simulink model "gm_UZ_EnDat_be4_segregation"  (R2023b)
settings: Solver=FixedStepAuto  StartTime=0  StopTime=0.000505  RelTol=1e-3
model workspace (MAT data in the model file):
  Select = 0
libraries: hdlsllib x74, simulink x21, hdlmdlgenlib x4, simulink_extras x1
(part 2 of 5)

== system gm_UZ_EnDat_be4_segregation/UZ_ENDAT/CLKDIV7 ==
  CLK1 : Inport  OutDataTypeStr=boolean  PortDimensions=1  SampleTime=1e-08
  Delay : Delay  DelayLength=double(1)  InitialCondition=0  SampleTime=1e-08
  Logical Operator1 : Logic  Operator=NOT  Inputs=1  AllPortsSameDT=off  OutDataTypeStr=boolean  SampleTime=1e-08
  Triggered Subsystem : Subsystem
  CLK/2 : Outport  OutDataTypeStr=boolean  SampleTime=1e-08  VectorParamsAs1DForOutWhenUnconnected=off
  wires:
  Logical Operator1/1 -> CLK/2/1, Delay/1
  Triggered Subsystem/1(Q) -> Logical Operator1/1
  CLK1/1 -> Triggered Subsystem/2(Trigger)
  Delay/1 -> Triggered Subsystem/1(D)

== system gm_UZ_EnDat_be4_segregation/UZ_ENDAT/CLKDIV8 ==
  CLK1 : Inport  OutDataTypeStr=boolean  PortDimensions=1  SampleTime=1e-08
  Delay : Delay  DelayLength=double(1)  InitialCondition=0  SampleTime=1e-08
  Logical Operator1 : Logic  Operator=NOT  Inputs=1  AllPortsSameDT=off  OutDataTypeStr=boolean  SampleTime=1e-08
  Triggered Subsystem : Subsystem
  CLK/2 : Outport  OutDataTypeStr=boolean  SampleTime=1e-08  VectorParamsAs1DForOutWhenUnconnected=off
  wires:
  Logical Operator1/1 -> CLK/2/1, Delay/1
  Triggered Subsystem/1(Q) -> Logical Operator1/1
  CLK1/1 -> Triggered Subsystem/2(Trigger)
  Delay/1 -> Triggered Subsystem/1(D)

== system gm_UZ_EnDat_be4_segregation/UZ_ENDAT/CLKDIV9 ==
  CLK1 : Inport  OutDataTypeStr=boolean  PortDimensions=1  SampleTime=1e-08
  Delay : Delay  DelayLength=double(1)  InitialCondition=0  SampleTime=1e-08
  Logical Operator1 : Logic  Operator=NOT  Inputs=1  AllPortsSameDT=off  OutDataTypeStr=boolean  SampleTime=1e-08
  Triggered Subsystem : Subsystem
  CLK/2 : Outport  OutDataTypeStr=boolean  SampleTime=1e-08  VectorParamsAs1DForOutWhenUnconnected=off
  wires:
  Logical Operator1/1 -> CLK/2/1, Delay/1
  Triggered Subsystem/1(Q) -> Logical Operator1/1
  CLK1/1 -> Triggered Subsystem/2(Trigger)
  Delay/1 -> Triggered Subsystem/1(D)

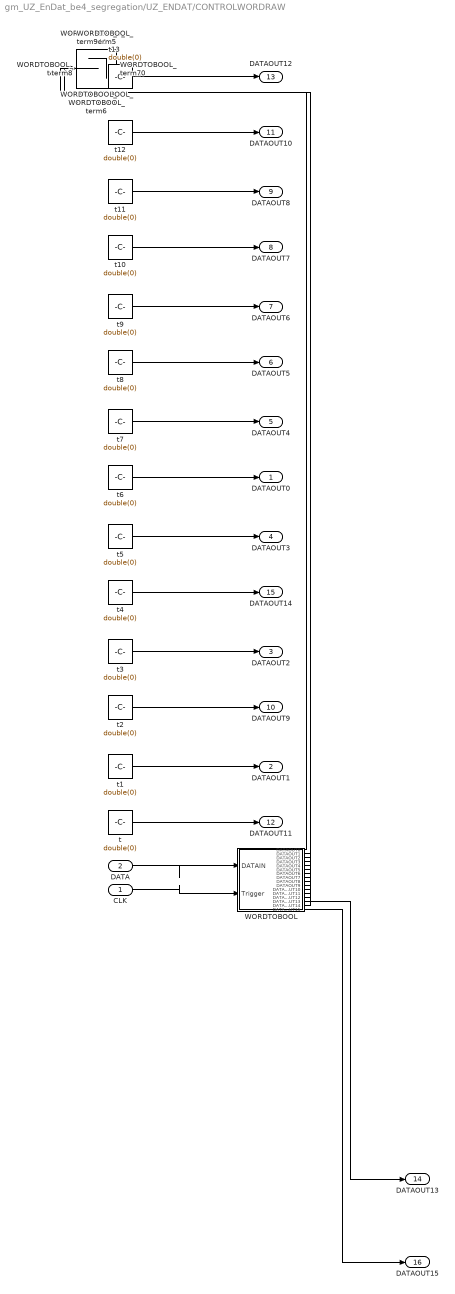
== system gm_UZ_EnDat_be4_segregation/UZ_ENDAT/CONTROLWORDRAW ==
  CLK : Inport  OutDataTypeStr=boolean  PortDimensions=1  SampleTime=1e-08
  DATA : Inport  Port=2  OutDataTypeStr=uint16  PortDimensions=1  SampleTime=1e-08
  WORDTOBOOL : Subsystem
  WORDTOBOOL_term{0..12,14} (14 alike) : Terminator
  t{,1..13} (14 alike) : Constant  Value=double(0)  OutDataTypeStr=boolean  SampleTime=1e-08
  DATAOUT0 : Outport  SampleTime=1e-08  VectorParamsAs1DForOutWhenUnconnected=off
  DATAOUT1 : Outport  Port=2  SampleTime=1e-08  VectorParamsAs1DForOutWhenUnconnected=off
  DATAOUT2 : Outport  Port=3  SampleTime=1e-08  VectorParamsAs1DForOutWhenUnconnected=off
  DATAOUT3 : Outport  Port=4  SampleTime=1e-08  VectorParamsAs1DForOutWhenUnconnected=off
  DATAOUT4 : Outport  Port=5  SampleTime=1e-08  VectorParamsAs1DForOutWhenUnconnected=off
  DATAOUT5 : Outport  Port=6  SampleTime=1e-08  VectorParamsAs1DForOutWhenUnconnected=off
  DATAOUT6 : Outport  Port=7  SampleTime=1e-08  VectorParamsAs1DForOutWhenUnconnected=off
  DATAOUT7 : Outport  Port=8  SampleTime=1e-08  VectorParamsAs1DForOutWhenUnconnected=off
  DATAOUT8 : Outport  Port=9  SampleTime=1e-08  VectorParamsAs1DForOutWhenUnconnected=off
  DATAOUT9 : Outport  Port=10  SampleTime=1e-08  VectorParamsAs1DForOutWhenUnconnected=off
  DATAOUT10 : Outport  Port=11  SampleTime=1e-08  VectorParamsAs1DForOutWhenUnconnected=off
  DATAOUT11 : Outport  Port=12  SampleTime=1e-08  VectorParamsAs1DForOutWhenUnconnected=off
  DATAOUT12 : Outport  Port=13  SampleTime=1e-08  VectorParamsAs1DForOutWhenUnconnected=off
  DATAOUT13 : Outport  Port=14  SampleTime=1e-08  VectorParamsAs1DForOutWhenUnconnected=off
  DATAOUT14 : Outport  Port=15  SampleTime=1e-08  VectorParamsAs1DForOutWhenUnconnected=off
  DATAOUT15 : Outport  Port=16  SampleTime=1e-08  VectorParamsAs1DForOutWhenUnconnected=off
  wires:
  CLK/1 -> WORDTOBOOL/2(Trigger)
  DATA/1 -> WORDTOBOOL/1(DATAIN)
  t6/1 -> DATAOUT0/1
  t1/1 -> DATAOUT1/1
  t3/1 -> DATAOUT2/1
  t5/1 -> DATAOUT3/1
  t7/1 -> DATAOUT4/1
  t8/1 -> DATAOUT5/1
  t9/1 -> DATAOUT6/1
  t10/1 -> DATAOUT7/1
  t11/1 -> DATAOUT8/1
  t2/1 -> DATAOUT9/1
  t12/1 -> DATAOUT10/1
  t/1 -> DATAOUT11/1
  t13/1 -> DATAOUT12/1
  WORDTOBOOL/14(DATAOUT13) -> DATAOUT13/1
  t4/1 -> DATAOUT14/1
  WORDTOBOOL/16(DATAOUT15) -> DATAOUT15/1
  WORDTOBOOL/1(DATAOUT0) -> WORDTOBOOL_term0/1
  WORDTOBOOL/2(DATAOUT1) -> WORDTOBOOL_term1/1
  WORDTOBOOL/3(DATAOUT2) -> WORDTOBOOL_term2/1
  WORDTOBOOL/4(DATAOUT3) -> WORDTOBOOL_term3/1
  WORDTOBOOL/5(DATAOUT4) -> WORDTOBOOL_term4/1
  WORDTOBOOL/6(DATAOUT5) -> WORDTOBOOL_term5/1
  WORDTOBOOL/7(DATAOUT6) -> WORDTOBOOL_term6/1
  WORDTOBOOL/8(DATAOUT7) -> WORDTOBOOL_term7/1
  WORDTOBOOL/9(DATAOUT8) -> WORDTOBOOL_term8/1
  WORDTOBOOL/10(DATAOUT9) -> WORDTOBOOL_term9/1
  WORDTOBOOL/11(DATAOUT10) -> WORDTOBOOL_term10/1
  WORDTOBOOL/12(DATAOUT11) -> WORDTOBOOL_term11/1
  WORDTOBOOL/13(DATAOUT12) -> WORDTOBOOL_term12/1
  WORDTOBOOL/15(DATAOUT14) -> WORDTOBOOL_term14/1

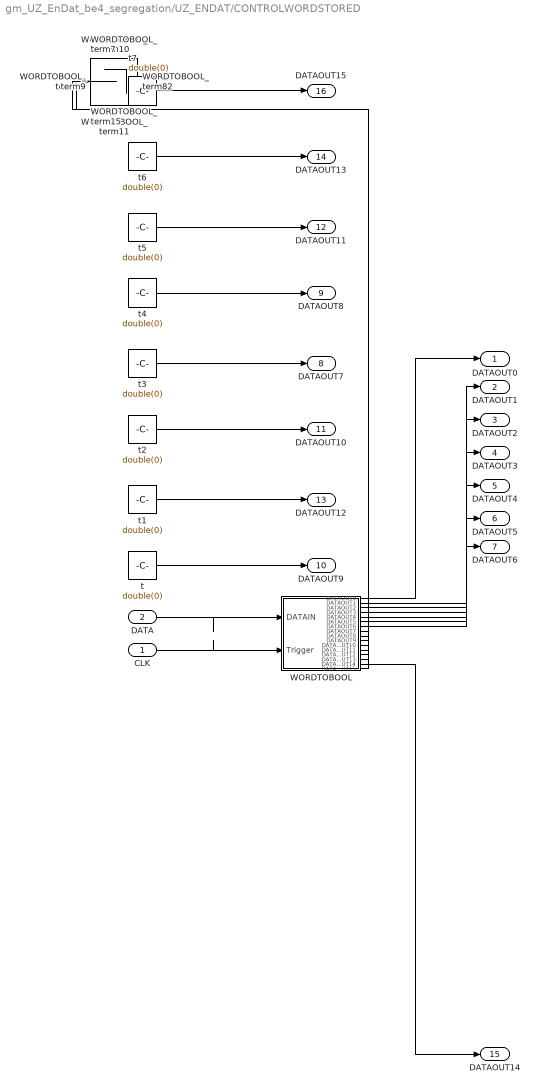
== system gm_UZ_EnDat_be4_segregation/UZ_ENDAT/CONTROLWORDSTORED ==
  CLK : Inport  OutDataTypeStr=boolean  PortDimensions=1  SampleTime=1e-08
  DATA : Inport  Port=2  OutDataTypeStr=uint16  PortDimensions=1  SampleTime=1e-08
  WORDTOBOOL : Subsystem
  WORDTOBOOL_term{7..13,15} (8 alike) : Terminator
  t{,1..7} (8 alike) : Constant  Value=double(0)  OutDataTypeStr=boolean  SampleTime=1e-08
  DATAOUT0 : Outport  SampleTime=1e-08  VectorParamsAs1DForOutWhenUnconnected=off
  DATAOUT1 : Outport  Port=2  SampleTime=1e-08  VectorParamsAs1DForOutWhenUnconnected=off
  DATAOUT2 : Outport  Port=3  SampleTime=1e-08  VectorParamsAs1DForOutWhenUnconnected=off
  DATAOUT3 : Outport  Port=4  SampleTime=1e-08  VectorParamsAs1DForOutWhenUnconnected=off
  DATAOUT4 : Outport  Port=5  SampleTime=1e-08  VectorParamsAs1DForOutWhenUnconnected=off
  DATAOUT5 : Outport  Port=6  SampleTime=1e-08  VectorParamsAs1DForOutWhenUnconnected=off
  DATAOUT6 : Outport  Port=7  SampleTime=1e-08  VectorParamsAs1DForOutWhenUnconnected=off
  DATAOUT7 : Outport  Port=8  SampleTime=1e-08  VectorParamsAs1DForOutWhenUnconnected=off
  DATAOUT8 : Outport  Port=9  SampleTime=1e-08  VectorParamsAs1DForOutWhenUnconnected=off
  DATAOUT9 : Outport  Port=10  SampleTime=1e-08  VectorParamsAs1DForOutWhenUnconnected=off
  DATAOUT10 : Outport  Port=11  SampleTime=1e-08  VectorParamsAs1DForOutWhenUnconnected=off
  DATAOUT11 : Outport  Port=12  SampleTime=1e-08  VectorParamsAs1DForOutWhenUnconnected=off
  DATAOUT12 : Outport  Port=13  SampleTime=1e-08  VectorParamsAs1DForOutWhenUnconnected=off
  DATAOUT13 : Outport  Port=14  SampleTime=1e-08  VectorParamsAs1DForOutWhenUnconnected=off
  DATAOUT14 : Outport  Port=15  SampleTime=1e-08  VectorParamsAs1DForOutWhenUnconnected=off
  DATAOUT15 : Outport  Port=16  SampleTime=1e-08  VectorParamsAs1DForOutWhenUnconnected=off
  wires:
  CLK/1 -> WORDTOBOOL/2(Trigger)
  DATA/1 -> WORDTOBOOL/1(DATAIN)
  WORDTOBOOL/1(DATAOUT0) -> DATAOUT0/1
  WORDTOBOOL/2(DATAOUT1) -> DATAOUT1/1
  WORDTOBOOL/3(DATAOUT2) -> DATAOUT2/1
  WORDTOBOOL/4(DATAOUT3) -> DATAOUT3/1
  WORDTOBOOL/5(DATAOUT4) -> DATAOUT4/1
  WORDTOBOOL/6(DATAOUT5) -> DATAOUT5/1
  WORDTOBOOL/7(DATAOUT6) -> DATAOUT6/1
  t3/1 -> DATAOUT7/1
  t4/1 -> DATAOUT8/1
  t/1 -> DATAOUT9/1
  t2/1 -> DATAOUT10/1
  t5/1 -> DATAOUT11/1
  t1/1 -> DATAOUT12/1
  t6/1 -> DATAOUT13/1
  WORDTOBOOL/15(DATAOUT14) -> DATAOUT14/1
  t7/1 -> DATAOUT15/1
  WORDTOBOOL/8(DATAOUT7) -> WORDTOBOOL_term7/1
  WORDTOBOOL/9(DATAOUT8) -> WORDTOBOOL_term8/1
  WORDTOBOOL/10(DATAOUT9) -> WORDTOBOOL_term9/1
  WORDTOBOOL/11(DATAOUT10) -> WORDTOBOOL_term10/1
  WORDTOBOOL/12(DATAOUT11) -> WORDTOBOOL_term11/1
  WORDTOBOOL/13(DATAOUT12) -> WORDTOBOOL_term12/1
  WORDTOBOOL/14(DATAOUT13) -> WORDTOBOOL_term13/1
  WORDTOBOOL/16(DATAOUT15) -> WORDTOBOOL_term15/1

== system gm_UZ_EnDat_be4_segregation/UZ_ENDAT/CRC_Check ==
  data : Inport  OutDataTypeStr=boolean  PortDimensions=1  SampleTime=1e-08
  set : Inport  Port=2  OutDataTypeStr=boolean  PortDimensions=1  SampleTime=1e-08
  clk : Inport  Port=3  OutDataTypeStr=boolean  PortDimensions=1  SampleTime=1e-08
  Constant : Constant  OutDataTypeStr=boolean  SampleTime=1e-08
  Constant1 : Constant  Value=0  OutDataTypeStr=boolean  SampleTime=1e-08
  FF0 : Subsystem
  FF0_term1 : Terminator
  FF1 : Subsystem
  FF1_term1 : Terminator
  FF2 : Subsystem
  FF2_term1 : Terminator
  FF3 : Subsystem
  FF3_term1 : Terminator
  FF4 : Subsystem
  Logical Operator : Logic  Operator=OR  AllPortsSameDT=off  OutDataTypeStr=boolean  SampleTime=1e-08
  Logical Operator{1..2,5..6} (4 alike) : Logic  AllPortsSameDT=off  OutDataTypeStr=boolean  SampleTime=1e-08
  Logical Operator3 : Logic  Operator=NOT  Inputs=1  AllPortsSameDT=off  OutDataTypeStr=boolean  SampleTime=1e-08
  Logical Operator4 : Logic  Operator=NOT  Inputs=1  AllPortsSameDT=off  OutDataTypeStr=boolean  SampleTime=1e-08
  Memory : UnitDelay  SampleTime=1e-08
  Memory1 : UnitDelay  SampleTime=1e-08
  Relational Operator : RelationalOperator  Operator===  OutDataTypeStr=boolean  SampleTime=1e-08  InputSameDT=off
  Relational Operator1 : RelationalOperator  Operator===  OutDataTypeStr=boolean  SampleTime=1e-08  InputSameDT=off
  Relational Operator2 : RelationalOperator  Operator===  OutDataTypeStr=boolean  SampleTime=1e-08  InputSameDT=off
  crc : Outport  SampleTime=1e-08
  wires:
  data/1 -> Logical Operator1/1, Relational Operator/2
  set/1 -> Logical Operator4/1, Logical Operator5/2, Logical Operator6/2
  clk/1 -> FF1/2(CLK), FF2/2(CLK), FF3/2(CLK), FF4/2(CLK), FF0/2(CLK)
  Constant/1 -> FF1/1(S), FF2/1(S), FF3/1(S), FF4/1(S), FF0/1(S)
  Constant1/1 -> FF1/4(R), FF2/4(R), FF3/4(R), FF4/4(R), FF0/4(R)
  FF0/2(NQ) -> FF0_term1/1
  FF1/2(NQ) -> FF1_term1/1
  FF2/2(NQ) -> FF2_term1/1
  FF3/2(NQ) -> FF3_term1/1
  FF4/2(NQ) -> Logical Operator2/1
  Logical Operator/1 -> crc/1
  Logical Operator1/1 -> Logical Operator/1
  Logical Operator2/1 -> Logical Operator/2
  Logical Operator3/1 -> Logical Operator1/2
  Logical Operator4/1 -> Logical Operator3/1, Logical Operator2/2
  Memory/1 -> Relational Operator1/2, Relational Operator2/2
  Logical Operator5/1 -> Memory1/1
  FF4/1(Q) -> Logical Operator5/1
  Logical Operator6/1 -> Memory/1
  Relational Operator/1 -> FF0/3(DATA), Logical Operator6/1
  Memory1/1 -> Relational Operator/1
  Relational Operator1/1 -> FF1/3(DATA)
  FF0/1(Q) -> Relational Operator1/1
  FF1/1(Q) -> FF2/3(DATA)
  Relational Operator2/1 -> FF3/3(DATA)
  FF2/1(Q) -> Relational Operator2/1
  FF3/1(Q) -> FF4/3(DATA)

== system gm_UZ_EnDat_be4_segregation/UZ_ENDAT/Compare To Constant ==
  u : Inport  OutDataTypeStr=fixdt(0,4,0,'DataTypeOverride', 'Off')  SampleTime=1e-08
  Compare : RelationalOperator  Operator===  OutDataTypeStr=boolean
  Constant : Constant  DisableCoverage=on  Value=const  OutDataTypeStr=Inherit: Inherit via back propagation  SampleTime=-1
  y : Outport  SampleTime=1e-08
  wires:
  u/1 -> Compare/1
  Compare/1 -> y/1
  Constant/1 -> Compare/2

== system gm_UZ_EnDat_be4_segregation/UZ_ENDAT/Compare To Constant1 ==
  u : Inport  OutDataTypeStr=fixdt(0,4,0,'DataTypeOverride', 'Off')  SampleTime=1e-08
  Compare : RelationalOperator  Operator===  OutDataTypeStr=boolean
  Constant : Constant  DisableCoverage=on  Value=const  OutDataTypeStr=Inherit: Inherit via back propagation  SampleTime=-1
  y : Outport  SampleTime=1e-08
  wires:
  u/1 -> Compare/1
  Compare/1 -> y/1
  Constant/1 -> Compare/2

== system gm_UZ_EnDat_be4_segregation/UZ_ENDAT/Compare To Constant2 ==
  u : Inport  OutDataTypeStr=fixdt(0,4,0,'DataTypeOverride', 'Off')  SampleTime=1e-08
  Compare : RelationalOperator  Operator===  OutDataTypeStr=boolean
  Constant : Constant  DisableCoverage=on  Value=const  OutDataTypeStr=Inherit: Inherit via back propagation  SampleTime=-1
  y : Outport  SampleTime=1e-08
  wires:
  u/1 -> Compare/1
  Compare/1 -> y/1
  Constant/1 -> Compare/2

== system gm_UZ_EnDat_be4_segregation/UZ_ENDAT/Data Type Conversion1 ==
  In1 : Inport
  Data Type Conversion1 : DataTypeConversion  OutDataTypeStr=double  SampleTime=1e-08  SaturateOnIntegerOverflow=off  RndMeth=Floor
  Data Type Conversion1_pd1 : Delay  DelayLength=3
  Out1 : Outport
  wires:
  In1/1 -> Data Type Conversion1/1
  Data Type Conversion1/1 -> Data Type Conversion1_pd1/1
  Data Type Conversion1_pd1/1 -> Out1/1

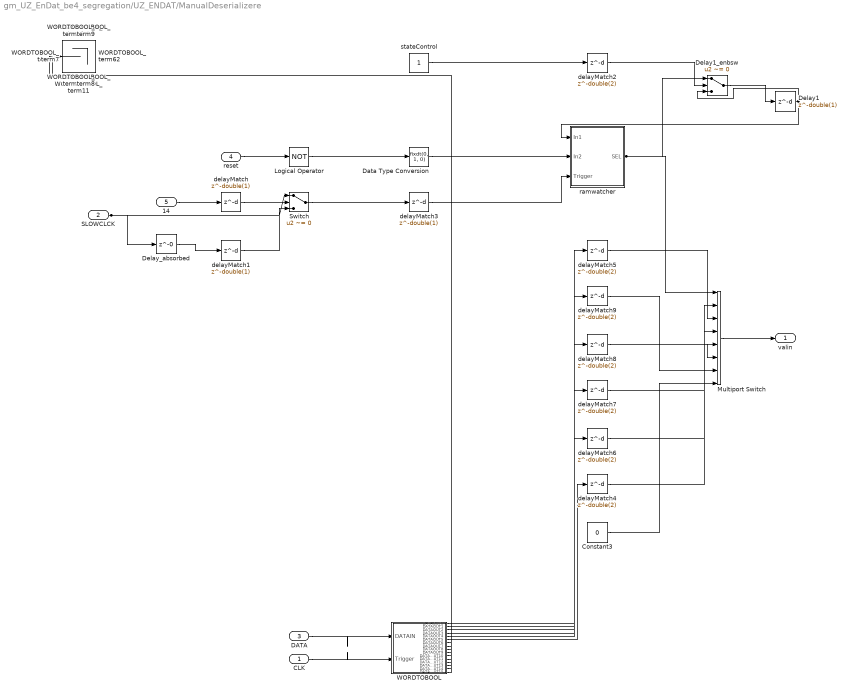
== system gm_UZ_EnDat_be4_segregation/UZ_ENDAT/ManualDeserializere ==
  CLK : Inport  OutDataTypeStr=boolean  PortDimensions=1  SampleTime=1e-08
  SLOWCLCK : Inport  Port=2  OutDataTypeStr=boolean  PortDimensions=1  SampleTime=1e-08
  DATA : Inport  Port=3  OutDataTypeStr=uint16  PortDimensions=1  SampleTime=1e-08
  reset : Inport  Port=4  OutDataTypeStr=boolean  PortDimensions=1  SampleTime=1e-08
  14 : Inport  Port=5  OutDataTypeStr=boolean  PortDimensions=1  SampleTime=1e-08
  Constant3 : Constant  Value=0  OutDataTypeStr=boolean  SampleTime=1e-08
  Data Type Conversion : DataTypeConversion  OutDataTypeStr=fixdt(0, 1, 0)  SampleTime=1e-08  SaturateOnIntegerOverflow=off  RndMeth=Floor
  Delay1 : Delay  DelayLength=double(1)  InitialCondition=0  SampleTime=1e-08
  Delay1_enbsw : Switch  Criteria=u2 ~= 0  Threshold=double(0)  OutDataTypeStr=uint16  SampleTime=1e-08  SaturateOnIntegerOverflow=off  InputSameDT=off
  Delay_absorbed : Delay  DelayLength=0
  Logical Operator : Logic  Operator=NOT  Inputs=1  AllPortsSameDT=off  OutDataTypeStr=boolean  SampleTime=1e-08
  Multiport Switch : MultiPortSwitch  Inputs=6  DataPortForDefault=Additional data port  DiagnosticForDefault=None  SampleTime=1e-08  SaturateOnIntegerOverflow=off  InputSameDT=off
  Switch : Switch  Criteria=u2 ~= 0  Threshold=double(0)  OutDataTypeStr=boolean  SampleTime=1e-08  SaturateOnIntegerOverflow=off  InputSameDT=off
  WORDTOBOOL : Subsystem
  WORDTOBOOL_term{6..15} (10 alike) : Terminator
  delayMatch : Delay  DelayLength=double(1)  InitialCondition=0  SampleTime=1e-08
  delayMatch1 : Delay  DelayLength=double(1)  InitialCondition=0  SampleTime=1e-08
  delayMatch{2,4..9} (7 alike) : Delay  DelayLength=double(2)  InitialCondition=0  SampleTime=1e-08
  delayMatch3 : Delay  DelayLength=double(1)  InitialCondition=0  SampleTime=1e-08
  ramwatcher : Subsystem
  stateControl : Constant  OutDataTypeStr=boolean  SampleTime=1e-08
  valin : Outport  SampleTime=1e-08
  wires:
  CLK/1 -> WORDTOBOOL/2(Trigger)
  SLOWCLCK/1 -> Switch/1, Delay_absorbed/1
  DATA/1 -> WORDTOBOOL/1(DATAIN)
  reset/1 -> Logical Operator/1
  delayMatch/1 -> Switch/2
  Constant3/1 -> Multiport Switch/8
  delayMatch1/1 -> Switch/3
  Logical Operator/1 -> Data Type Conversion/1
  Multiport Switch/1 -> valin/1
  delayMatch9/1 -> Multiport Switch/7
  delayMatch8/1 -> Multiport Switch/6
  delayMatch7/1 -> Multiport Switch/5
  delayMatch6/1 -> Multiport Switch/4
  delayMatch5/1 -> Multiport Switch/3
  delayMatch4/1 -> Multiport Switch/2
  WORDTOBOOL/7(DATAOUT6) -> WORDTOBOOL_term6/1
  WORDTOBOOL/8(DATAOUT7) -> WORDTOBOOL_term7/1
  WORDTOBOOL/9(DATAOUT8) -> WORDTOBOOL_term8/1
  WORDTOBOOL/10(DATAOUT9) -> WORDTOBOOL_term9/1
  WORDTOBOOL/11(DATAOUT10) -> WORDTOBOOL_term10/1
  WORDTOBOOL/12(DATAOUT11) -> WORDTOBOOL_term11/1
  WORDTOBOOL/13(DATAOUT12) -> WORDTOBOOL_term12/1
  WORDTOBOOL/14(DATAOUT13) -> WORDTOBOOL_term13/1
  WORDTOBOOL/15(DATAOUT14) -> WORDTOBOOL_term14/1
  WORDTOBOOL/16(DATAOUT15) -> WORDTOBOOL_term15/1
  14/1 -> delayMatch/1
  Delay_absorbed/1 -> delayMatch1/1
  stateControl/1 -> delayMatch2/1
  Switch/1 -> delayMatch3/1
  WORDTOBOOL/6(DATAOUT5) -> delayMatch4/1
  WORDTOBOOL/5(DATAOUT4) -> delayMatch5/1
  WORDTOBOOL/4(DATAOUT3) -> delayMatch6/1
  WORDTOBOOL/3(DATAOUT2) -> delayMatch7/1
  WORDTOBOOL/2(DATAOUT1) -> delayMatch8/1
  WORDTOBOOL/1(DATAOUT0) -> delayMatch9/1
  ramwatcher/1(SEL) -> Delay1_enbsw/1, Multiport Switch/1
  Data Type Conversion/1 -> ramwatcher/2(In2)
  delayMatch3/1 -> ramwatcher/3(Trigger)
  delayMatch2/1 -> Delay1_enbsw/2
  Delay1/1 -> Delay1_enbsw/3, ramwatcher/1(In1)
  Delay1_enbsw/1 -> Delay1/1

== system gm_UZ_EnDat_be4_segregation/UZ_ENDAT/ManualSerialize ==
  CLK : Inport  OutDataTypeStr=boolean  PortDimensions=1  SampleTime=1e-08
  SLOWCLCK : Inport  Port=2  OutDataTypeStr=boolean  PortDimensions=1  SampleTime=1e-08
  DATA : Inport  Port=3  OutDataTypeStr=boolean  PortDimensions=1  SampleTime=1e-08
  recieving : Inport  Port=4  OutMin=0  OutMax=1  OutDataTypeStr=boolean  PortDimensions=1  SampleTime=1e-08
  recievecnt : Inport  Port=5  OutDataTypeStr=uint16  PortDimensions=1  SampleTime=1e-08
  CLKCNTER_RECIEVE : Subsystem
  Logical Operator : Logic  Operator=NOT  Inputs=1  AllPortsSameDT=off  OutDataTypeStr=boolean  SampleTime=1e-08
  Logical Operator3 : Logic  AllPortsSameDT=off  OutDataTypeStr=boolean  SampleTime=1e-08
  Memory : UnitDelay  InitialCondition="fi(0,0,64,0,\"hex\",\"0000000000000000\")"  SampleTime=1e-08
  Memory_enbsw : Switch  Criteria=u2 ~= 0  Threshold=double(0)  OutDataTypeStr=fixdt(0, 64, 0)  SampleTime=1e-08  SaturateOnIntegerOverflow=off  InputSameDT=off
  Relational Operator : RelationalOperator  Operator===  OutDataTypeStr=boolean  SampleTime=1e-08  InputSameDT=off
  SetZero64 : Subsystem
  Storage16 : Subsystem
  Triggered Subsystem : Subsystem
  delayMatch{,1..3} (4 alike) : Delay  DelayLength=double(2)  InitialCondition=0  SampleTime=1e-08
  stateControl : Constant  OutDataTypeStr=boolean  SampleTime=1e-08
  valueout : Outport  OutDataTypeStr=uint64  SampleTime=1e-08
  wrok : Outport  Port=2  OutDataTypeStr=boolean  SampleTime=1e-08
  wires:
  SLOWCLCK/1 -> Logical Operator3/1, CLKCNTER_RECIEVE/2(CLK2CNT)
  recieving/1 -> Logical Operator3/2, Logical Operator/1
  delayMatch3/1 -> Relational Operator/2
  CLKCNTER_RECIEVE/1(CNT) -> Relational Operator/1
  Logical Operator/1 -> CLKCNTER_RECIEVE/3(ResetCNT), SetZero64/2(setzero)
  Relational Operator/1 -> Storage16/2(Write)
  Storage16/1(out) -> valueout/1
  Storage16/2(wrok) -> wrok/1
  stateControl/1 -> delayMatch/1
  DATA/1 -> delayMatch1/1
  CLK/1 -> delayMatch2/1, CLKCNTER_RECIEVE/1(CLK)
  recievecnt/1 -> delayMatch3/1
  SetZero64/1(valueout) -> Memory_enbsw/1, Storage16/1(Data)
  delayMatch1/1 -> Triggered Subsystem/1(In1)
  Logical Operator3/1 -> Triggered Subsystem/3(Trigger)
  delayMatch2/1 -> SetZero64/3(Trigger)
  Triggered Subsystem/1(valin) -> SetZero64/1(valin)
  delayMatch/1 -> Memory_enbsw/2
  Memory/1 -> Memory_enbsw/3, Triggered Subsystem/2(valueout)
  Memory_enbsw/1 -> Memory/1

== system gm_UZ_EnDat_be4_segregation/UZ_ENDAT/OUTPUTCONTROLCONTINIOUS ==
  CLKCNT : Inport  OutDataTypeStr=uint32  PortDimensions=1  SampleTime=1e-08
  CLKS2DATAFLOWCHG : Inport  Port=2  OutDataTypeStr=uint8  PortDimensions=1  SampleTime=1e-08
  CLK2ENDOFTRANSMISSION : Inport  Port=3  OutDataTypeStr=uint16  PortDimensions=1  SampleTime=1e-08
  OPENCOM : Inport  Port=4  OutDataTypeStr=boolean  PortDimensions=1  SampleTime=1e-08
  Logical Operator : Logic  Operator=OR  AllPortsSameDT=off  OutDataTypeStr=boolean  SampleTime=1e-08
  Logical Operator6 : Logic  Operator=NOT  Inputs=1  AllPortsSameDT=off  OutDataTypeStr=boolean  SampleTime=1e-08
  Relational Operator : RelationalOperator  Operator=<=  OutDataTypeStr=boolean  SampleTime=1e-08  InputSameDT=off
  Relational Operator1 : RelationalOperator  OutDataTypeStr=boolean  SampleTime=1e-08  InputSameDT=off
  CLKOFF : Outport  OutDataTypeStr=boolean  SampleTime=1e-08
  DATAINV : Outport  Port=2  OutDataTypeStr=boolean  SampleTime=1e-08
  RESETCNT : Outport  Port=3  OutDataTypeStr=boolean  SampleTime=1e-08
  wires:
  CLKCNT/1 -> Relational Operator1/1, Relational Operator/1
  CLKS2DATAFLOWCHG/1 -> Relational Operator/2
  CLK2ENDOFTRANSMISSION/1 -> Relational Operator1/2
  OPENCOM/1 -> Logical Operator6/1
  Logical Operator/1 -> CLKOFF/1
  Logical Operator6/1 -> Logical Operator/1
  Relational Operator/1 -> DATAINV/1
  Relational Operator1/1 -> Logical Operator/2, RESETCNT/1

== system gm_UZ_EnDat_be4_segregation/UZ_ENDAT/RECOVERYTIME ==
  in0 : Inport  OutDataTypeStr=boolean  SampleTime=1e-08
  stateControl_enb : EnablePort  OutDataTypeStr=boolean
  RECOVERYTIME : simulink/Discrete/Tapped Delay  vinit=0  samptime=-1  NumDelays=double(2000)  DelayOrder=Newest  includeCurrent=on
  out0 : Outport  OutDataTypeStr=boolean  PortDimensions=[2001]  SampleTime=1e-08
  wires:
  RECOVERYTIME/1 -> out0/1
  in0/1 -> RECOVERYTIME/1

== system gm_UZ_EnDat_be4_segregation/UZ_ENDAT/SetZero ==
  valin : Inport  OutDataTypeStr=fixdt(0, 2, 0)  PortDimensions=1  SampleTime=1e-08
  setzero : Inport  Port=2  OutDataTypeStr=boolean  PortDimensions=1  SampleTime=1e-08
  Trigger : Inport  Port=3  OutDataTypeStr=boolean  SampleTime=1e-08
  Constant1 : Constant  OutDataTypeStr=fixdt(0, 2, 0)  SampleTime=1e-08
  Constant2 : Constant  Value=0  OutDataTypeStr=fixdt(0, 2, 0)  SampleTime=1e-08
  Index Vector1 : MultiPortSwitch  DataPortOrder=Zero-based contiguous  Inputs=2  DiagnosticForDefault=None  zeroidx=on  OutDataTypeStr=fixdt(0, 2, 0)  SampleTime=1e-08  SaturateOnIntegerOverflow=off  InputSameDT=off
  PipelineRegister : Delay  DelayLength=double(1)  InitialCondition=0
  Product : Product  Inputs=**  OutDataTypeStr=fixdt(0, 4, 0)  SampleTime=1e-08
  Product_out1bypassMux : MultiPortSwitch  DataPortOrder=Zero-based contiguous  Inputs=2  zeroidx=on  OutDataTypeStr=fixdt(0, 4, 0)  SampleTime=1e-08  SaturateOnIntegerOverflow=off  InputSameDT=off
  Trigger_delay : Delay  DelayLength=double(1)  InitialCondition=0
  Trigger_delay_Initial_Val : Constant  OutDataTypeStr=boolean  SampleTime=1e-08
  Trigger_delay_ctrl_const : Constant  OutDataTypeStr=boolean  SampleTime=1e-08
  Trigger_delay_ctrl_delay : Delay  DelayLength=double(1)  InitialCondition=0
  Trigger_delay_switch : Switch  Criteria=u2 ~= 0  Threshold=double(0)  OutDataTypeStr=boolean  SampleTime=1e-08  SaturateOnIntegerOverflow=off  InputSameDT=off
  Trigger_delayed_inverted_and_Trigger : Logic  AllPortsSameDT=off  OutDataTypeStr=boolean  SampleTime=1e-08
  delayMatch : Delay  DelayLength=double(1)  InitialCondition=0
  delayMatch1 : Delay  DelayLength=double(1)  InitialCondition=0
  delayMatch2 : Delay  DelayLength=double(1)  InitialCondition=0
  not_Trigger_delayed : Logic  Operator=NOT  Inputs=1  AllPortsSameDT=off  OutDataTypeStr=boolean  SampleTime=1e-08
  out0_bypass : UnitDelay  InitialCondition=double(0)  SampleTime=1e-08
  out0_bypass_Initial_Val : Constant  OutDataTypeStr=fixdt(0, 4, 0)  SampleTime=1e-08
  out0_bypass_ctrl_const : Constant  OutDataTypeStr=boolean  SampleTime=1e-08
  out0_bypass_ctrl_delay : Delay  DelayLength=double(1)  InitialCondition=0
  out0_bypass_switch : Switch  Criteria=u2 ~= 0  Threshold=double(0)  OutDataTypeStr=fixdt(0, 4, 0)  SampleTime=1e-08  SaturateOnIntegerOverflow=off  InputSameDT=off
  valueout : Outport  SampleTime=1e-08  InitialOutput=0  VectorParamsAs1DForOutWhenUnconnected=off
  wires:
  Trigger/1 -> Trigger_delayed_inverted_and_Trigger/2, Trigger_delay/1
  valin/1 -> Product/2
  setzero/1 -> Index Vector1/1
  Trigger_delay_switch/1 -> not_Trigger_delayed/1
  not_Trigger_delayed/1 -> Trigger_delayed_inverted_and_Trigger/1
  Trigger_delay/1 -> Trigger_delay_switch/1
  Trigger_delay_Initial_Val/1 -> Trigger_delay_switch/3
  Trigger_delay_ctrl_const/1 -> Trigger_delay_ctrl_delay/1
  Trigger_delay_ctrl_delay/1 -> Trigger_delay_switch/2
  Index Vector1/1 -> Product/1
  Constant1/1 -> Index Vector1/2
  Constant2/1 -> Index Vector1/3
  out0_bypass_ctrl_const/1 -> out0_bypass_ctrl_delay/1
  out0_bypass_ctrl_delay/1 -> delayMatch/1
  out0_bypass_Initial_Val/1 -> delayMatch1/1
  Trigger_delayed_inverted_and_Trigger/1 -> delayMatch2/1
  Product_out1bypassMux/1 -> out0_bypass/1, valueout/1
  out0_bypass/1 -> out0_bypass_switch/1
  delayMatch/1 -> out0_bypass_switch/2
  delayMatch1/1 -> out0_bypass_switch/3
  delayMatch2/1 -> Product_out1bypassMux/1
  PipelineRegister/1 -> Product_out1bypassMux/3
  out0_bypass_switch/1 -> Product_out1bypassMux/2
  Product/1 -> PipelineRegister/1

== system gm_UZ_EnDat_be4_segregation/UZ_ENDAT/SetZeroBool ==
  valin : Inport  OutDataTypeStr=boolean  PortDimensions=1  SampleTime=1e-08
  setzero : Inport  Port=2  OutDataTypeStr=boolean  PortDimensions=1  SampleTime=1e-08
  Trigger : Inport  Port=3  OutDataTypeStr=boolean  SampleTime=1e-08
  Constant1 : Constant  OutDataTypeStr=boolean  SampleTime=1e-08
  Constant2 : Constant  Value=0  OutDataTypeStr=boolean  SampleTime=1e-08
  Index Vector1 : MultiPortSwitch  DataPortOrder=Zero-based contiguous  Inputs=2  DiagnosticForDefault=None  zeroidx=on  SampleTime=1e-08  SaturateOnIntegerOverflow=off  InputSameDT=off
  Logical Operator : Logic  AllPortsSameDT=off  OutDataTypeStr=boolean  SampleTime=1e-08
  Logical Operator_out1bypassMux : MultiPortSwitch  DataPortOrder=Zero-based contiguous  Inputs=2  zeroidx=on  SampleTime=1e-08  SaturateOnIntegerOverflow=off  InputSameDT=off
  Trigger_delay : Delay  DelayLength=double(1)  InitialCondition=0
  Trigger_delay_Initial_Val : Constant  OutDataTypeStr=boolean  SampleTime=1e-08
  Trigger_delay_ctrl_const : Constant  OutDataTypeStr=boolean  SampleTime=1e-08
  Trigger_delay_ctrl_delay : Delay  DelayLength=double(1)  InitialCondition=0
  Trigger_delay_switch : Switch  Criteria=u2 ~= 0  Threshold=double(0)  OutDataTypeStr=boolean  SampleTime=1e-08  SaturateOnIntegerOverflow=off  InputSameDT=off
  Trigger_delayed_inverted_and_Trigger : Logic  AllPortsSameDT=off  OutDataTypeStr=boolean  SampleTime=1e-08
  delayMatch{,1..5} (6 alike) : Delay  DelayLength=double(2)  InitialCondition=0
  not_Trigger_delayed : Logic  Operator=NOT  Inputs=1  AllPortsSameDT=off  OutDataTypeStr=boolean  SampleTime=1e-08
  out0_bypass : UnitDelay  InitialCondition=double(0)  SampleTime=1e-08
  out0_bypass_Initial_Val : Constant  OutDataTypeStr=boolean  SampleTime=1e-08
  out0_bypass_ctrl_const : Constant  OutDataTypeStr=boolean  SampleTime=1e-08
  out0_bypass_ctrl_delay : Delay  DelayLength=double(1)  InitialCondition=0
  out0_bypass_switch : Switch  Criteria=u2 ~= 0  Threshold=double(0)  OutDataTypeStr=boolean  SampleTime=1e-08  SaturateOnIntegerOverflow=off  InputSameDT=off
  valueout : Outport  SampleTime=1e-08  InitialOutput=0  VectorParamsAs1DForOutWhenUnconnected=off
  wires:
  Trigger/1 -> Trigger_delayed_inverted_and_Trigger/2, Trigger_delay/1
  valin/1 -> Logical Operator/2
  setzero/1 -> Index Vector1/1
  Trigger_delay_switch/1 -> not_Trigger_delayed/1
  not_Trigger_delayed/1 -> Trigger_delayed_inverted_and_Trigger/1
  Trigger_delay/1 -> Trigger_delay_switch/1
  delayMatch1/1 -> Trigger_delay_switch/3
  delayMatch/1 -> Trigger_delay_switch/2
  Index Vector1/1 -> Logical Operator/1
  delayMatch2/1 -> Index Vector1/2
  delayMatch3/1 -> Index Vector1/3
  Trigger_delay_ctrl_delay/1 -> delayMatch/1
  Trigger_delay_Initial_Val/1 -> delayMatch1/1
  Constant1/1 -> delayMatch2/1
  Constant2/1 -> delayMatch3/1
  out0_bypass_ctrl_delay/1 -> delayMatch4/1
  out0_bypass_Initial_Val/1 -> delayMatch5/1
  Logical Operator_out1bypassMux/1 -> out0_bypass/1, valueout/1
  out0_bypass/1 -> out0_bypass_switch/1
  delayMatch4/1 -> out0_bypass_switch/2
  delayMatch5/1 -> out0_bypass_switch/3
  Trigger_delayed_inverted_and_Trigger/1 -> Logical Operator_out1bypassMux/1
  Logical Operator/1 -> Logical Operator_out1bypassMux/3
  out0_bypass_switch/1 -> Logical Operator_out1bypassMux/2
  out0_bypass_ctrl_const/1 -> out0_bypass_ctrl_delay/1
  Trigger_delay_ctrl_const/1 -> Trigger_delay_ctrl_delay/1

== system gm_UZ_EnDat_be4_segregation/UZ_ENDAT/SetZeroBool1 ==
  valin : Inport  OutDataTypeStr=boolean  PortDimensions=1  SampleTime=1e-08
  setzero : Inport  Port=2  OutDataTypeStr=boolean  PortDimensions=1  SampleTime=1e-08
  Trigger : Inport  Port=3  OutDataTypeStr=boolean  SampleTime=1e-08
  Constant1 : Constant  OutDataTypeStr=boolean  SampleTime=1e-08
  Constant2 : Constant  Value=0  OutDataTypeStr=boolean  SampleTime=1e-08
  Index Vector1 : MultiPortSwitch  DataPortOrder=Zero-based contiguous  Inputs=2  DiagnosticForDefault=None  zeroidx=on  SampleTime=1e-08  SaturateOnIntegerOverflow=off  InputSameDT=off
  Logical Operator : Logic  AllPortsSameDT=off  OutDataTypeStr=boolean  SampleTime=1e-08
  Logical Operator_out1bypassMux : MultiPortSwitch  DataPortOrder=Zero-based contiguous  Inputs=2  zeroidx=on  SampleTime=1e-08  SaturateOnIntegerOverflow=off  InputSameDT=off
  Trigger_delay : Delay  DelayLength=double(1)  InitialCondition=0
  Trigger_delay_Initial_Val : Constant  OutDataTypeStr=boolean  SampleTime=1e-08
  Trigger_delay_ctrl_const : Constant  OutDataTypeStr=boolean  SampleTime=1e-08
  Trigger_delay_ctrl_delay : Delay  DelayLength=double(1)  InitialCondition=0
  Trigger_delay_switch : Switch  Criteria=u2 ~= 0  Threshold=double(0)  OutDataTypeStr=boolean  SampleTime=1e-08  SaturateOnIntegerOverflow=off  InputSameDT=off
  Trigger_delayed_inverted_and_Trigger : Logic  AllPortsSameDT=off  OutDataTypeStr=boolean  SampleTime=1e-08
  delayMatch : Delay  DelayLength=double(2)  InitialCondition=0
  delayMatch1 : Delay  DelayLength=double(2)  InitialCondition=0
  delayMatch2 : Delay  DelayLength=double(2)  InitialCondition=0
  not_Trigger_delayed : Logic  Operator=NOT  Inputs=1  AllPortsSameDT=off  OutDataTypeStr=boolean  SampleTime=1e-08
  out0_bypass : UnitDelay  InitialCondition=double(0)  SampleTime=1e-08
  out0_bypass_Initial_Val : Constant  OutDataTypeStr=boolean  SampleTime=1e-08
  out0_bypass_ctrl_const : Constant  OutDataTypeStr=boolean  SampleTime=1e-08
  out0_bypass_ctrl_delay : Delay  DelayLength=double(1)  InitialCondition=0
  out0_bypass_switch : Switch  Criteria=u2 ~= 0  Threshold=double(0)  OutDataTypeStr=boolean  SampleTime=1e-08  SaturateOnIntegerOverflow=off  InputSameDT=off
  valueout : Outport  SampleTime=1e-08  InitialOutput=0  VectorParamsAs1DForOutWhenUnconnected=off
  wires:
  Trigger/1 -> Trigger_delayed_inverted_and_Trigger/2, Trigger_delay/1
  valin/1 -> Logical Operator/2
  setzero/1 -> Index Vector1/1
  Trigger_delay_switch/1 -> not_Trigger_delayed/1
  not_Trigger_delayed/1 -> Trigger_delayed_inverted_and_Trigger/1
  Trigger_delay/1 -> Trigger_delay_switch/1
  Trigger_delay_Initial_Val/1 -> Trigger_delay_switch/3
  Trigger_delay_ctrl_const/1 -> Trigger_delay_ctrl_delay/1
  Trigger_delay_ctrl_delay/1 -> Trigger_delay_switch/2
  Index Vector1/1 -> Logical Operator/1
  Constant1/1 -> Index Vector1/2
  Constant2/1 -> Index Vector1/3
  out0_bypass_ctrl_const/1 -> out0_bypass_ctrl_delay/1
  out0_bypass_ctrl_delay/1 -> delayMatch/1
  out0_bypass_Initial_Val/1 -> delayMatch1/1
  Trigger_delayed_inverted_and_Trigger/1 -> delayMatch2/1
  Logical Operator_out1bypassMux/1 -> out0_bypass/1, valueout/1
  out0_bypass/1 -> out0_bypass_switch/1
  delayMatch/1 -> out0_bypass_switch/2
  delayMatch1/1 -> out0_bypass_switch/3
  delayMatch2/1 -> Logical Operator_out1bypassMux/1
  Logical Operator/1 -> Logical Operator_out1bypassMux/3
  out0_bypass_switch/1 -> Logical Operator_out1bypassMux/2

== system gm_UZ_EnDat_be4_segregation/UZ_ENDAT/Storage16 ==
  Data : Inport  OutDataTypeStr=uint16  PortDimensions=1  SampleTime=1e-08
  Write : Inport  Port=2  OutDataTypeStr=boolean  PortDimensions=1  SampleTime=1e-08
  Compare To Zero : Subsystem  mask(Compare To Zero){relop===, OutDataTypeStr=boolean, ZeroCross=on}
      mask prompts: relop "Simulink:masks:Operator_MP"; OutDataTypeStr "Simulink:masks:OutputDataType_MP"; ZeroCross "Simulink:masks:EnableZerocrossingDetection_MP"
      mask help: Simulink:masks:CompareToZero_MD
      mask init:
      | OutDataTypeStr = 'boolean';
      | ZeroCross = 'on';
      | blkName = 'UZ_EnDat_be4_segregation/UZ_ENDAT/Storage16/Compare\nTo Zero';
      | relop = '==';
      | setValue = 'boolean';
      mask TypeOptions relop: == | ~= | < | <= | >= | >
      mask TypeOptions OutDataTypeStr: Simulink:masks:uint8 | Simulink:masks:boolean
      mask Callback ZeroCross: sl('zeroCrossEnable', gcbh);
      mask Display: disp([relop,' 0'])
  Logical Operator : Logic  Operator=NOT  Inputs=1  AllPortsSameDT=off  OutDataTypeStr=boolean  SampleTime=1e-08
  Logical Operator1 : Logic  Inputs=3  AllPortsSameDT=off  OutDataTypeStr=boolean  SampleTime=1e-08
  Logical Operator2 : Logic  Operator=NOT  Inputs=1  AllPortsSameDT=off  OutDataTypeStr=boolean  SampleTime=1e-08
  Logical Operator3 : Logic  AllPortsSameDT=off  OutDataTypeStr=boolean  SampleTime=1e-08
  Relational Operator : RelationalOperator  Operator===  OutDataTypeStr=boolean  SampleTime=1e-08  InputSameDT=off
  Single Port RAM System : hdlsllib/HDL RAMs/Single Port RAM System  RAMType=Single port  AsyncRead=off  WriteOutputValue=Old data  RAMInitialValue=0  allowBusInputs=off  WritesHaveOutput=on  NumReads=0  NumWrites=1  SimulateUsing=Code generation
  adress : Constant  Value=5  OutDataTypeStr=uint8  SampleTime=1e-08
  out : Outport  SampleTime=1e-08
  wrok : Outport  Port=2  OutDataTypeStr=boolean  SampleTime=1e-08
  wires:
  Data/1 -> Compare To Zero/1(u), Relational Operator/2, Single Port RAM System/1
  Write/1 -> Logical Operator1/1
  Compare To Zero/1(y) -> Logical Operator2/1
  Logical Operator2/1 -> Logical Operator3/2, Logical Operator1/3
  Logical Operator3/1 -> wrok/1
  Relational Operator/1 -> Logical Operator3/1, Logical Operator/1
  Single Port RAM System/1 -> out/1, Relational Operator/1
  adress/1 -> Single Port RAM System/2
  Logical Operator/1 -> Logical Operator1/2
  Logical Operator1/1 -> Single Port RAM System/3

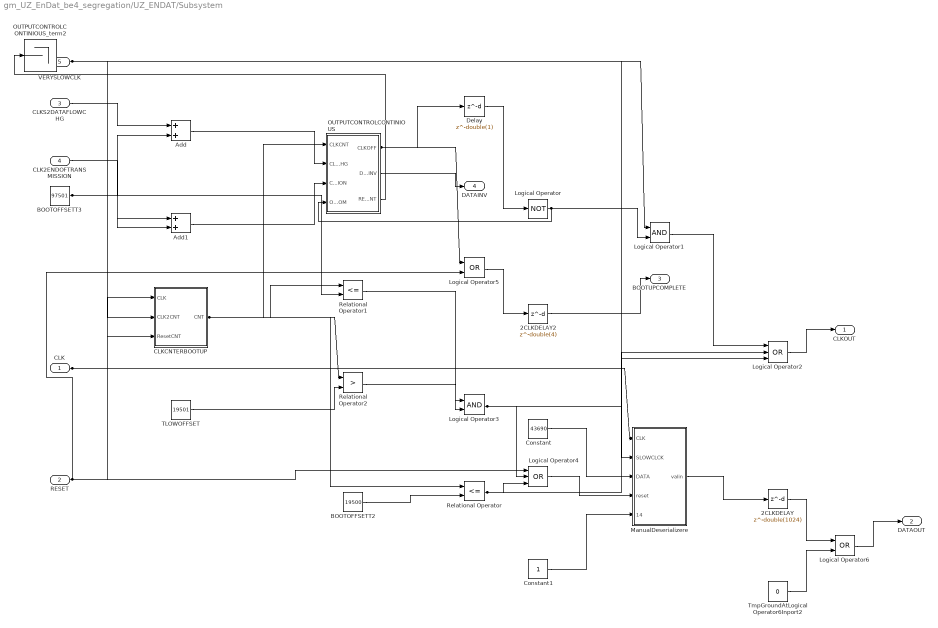
== system gm_UZ_EnDat_be4_segregation/UZ_ENDAT/Subsystem ==
  CLK : Inport  OutDataTypeStr=boolean  PortDimensions=1  SampleTime=1e-08
  RESET : Inport  Port=2  OutDataTypeStr=boolean  PortDimensions=1  SampleTime=1e-08
  CLKS2DATAFLOWCHG : Inport  Port=3  OutDataTypeStr=uint8  PortDimensions=1  SampleTime=1e-08
  CLK2ENDOFTRANSMISSION : Inport  Port=4  OutDataTypeStr=uint16  PortDimensions=1  SampleTime=1e-08
  VERYSLOWCLK : Inport  Port=5  OutDataTypeStr=boolean  PortDimensions=1  SampleTime=1e-08
  2CLKDELAY : Delay  DelayLength=double(1024)  InitialCondition=0  SampleTime=1e-08
  2CLKDELAY2 : Delay  DelayLength=double(4)  InitialCondition=0  SampleTime=1e-08
  Add : Sum  OutDataTypeStr=uint32  AccumDataTypeStr=uint32  SampleTime=1e-08
  Add1 : Sum  OutDataTypeStr=uint32  AccumDataTypeStr=uint32  SampleTime=1e-08
  BOOTOFFSETT2 : Constant  Value=19500  OutDataTypeStr=uint32  SampleTime=1e-08
  BOOTOFFSETT3 : Constant  Value=97501  OutDataTypeStr=uint32  SampleTime=1e-08
  CLKCNTERBOOTUP : Subsystem
  Constant : Constant  Value=43690  OutDataTypeStr=uint16  SampleTime=1e-08
  Constant1 : Constant  OutDataTypeStr=boolean  SampleTime=1e-08
  Delay : Delay  DelayLength=double(1)  InitialCondition=0  SampleTime=1e-08
  Logical Operator : Logic  Operator=NOT  Inputs=1  AllPortsSameDT=off  OutDataTypeStr=boolean  SampleTime=1e-08
  Logical Operator1 : Logic  AllPortsSameDT=off  OutDataTypeStr=boolean  SampleTime=1e-08
  Logical Operator2 : Logic  Operator=OR  Inputs=3  AllPortsSameDT=off  OutDataTypeStr=boolean  SampleTime=1e-08
  Logical Operator3 : Logic  AllPortsSameDT=off  OutDataTypeStr=boolean  SampleTime=1e-08
  Logical Operator4 : Logic  Operator=OR  Inputs=3  AllPortsSameDT=off  OutDataTypeStr=boolean  SampleTime=1e-08
  Logical Operator5 : Logic  Operator=OR  AllPortsSameDT=off  OutDataTypeStr=boolean  SampleTime=1e-08
  Logical Operator6 : Logic  Operator=OR  AllPortsSameDT=off  OutDataTypeStr=boolean  SampleTime=1e-08
  ManualDeserializere : Subsystem
  OUTPUTCONTROLCONTINIOUS : Subsystem
  OUTPUTCONTROLCONTINIOUS_term2 : Terminator
  Relational Operator : RelationalOperator  Operator=<=  OutDataTypeStr=boolean  SampleTime=1e-08  InputSameDT=off
  Relational Operator1 : RelationalOperator  Operator=<=  OutDataTypeStr=boolean  SampleTime=1e-08  InputSameDT=off
  Relational Operator2 : RelationalOperator  Operator=>  OutDataTypeStr=boolean  SampleTime=1e-08  InputSameDT=off
  TLOWOFFSET : Constant  Value=19501  OutDataTypeStr=uint32  SampleTime=1e-08
  TmpGroundAtLogical Operator6Inport2 : Constant  Value=0  VectorParams1D=off  OutDataTypeStr=boolean  SampleTime=1e-08
  CLKOUT : Outport  SampleTime=1e-08
  DATAOUT : Outport  Port=2  SampleTime=1e-08
  BOOTUPCOMPLETE : Outport  Port=3  OutDataTypeStr=boolean  SampleTime=1e-08
  DATAINV : Outport  Port=4  SampleTime=1e-08
  wires:
  CLK/1 -> CLKCNTERBOOTUP/1(CLK), ManualDeserializere/1(CLK)
  RESET/1 -> Logical Operator5/2, Logical Operator4/1, CLKCNTERBOOTUP/3(ResetCNT)
  CLKS2DATAFLOWCHG/1 -> Add/1
  CLK2ENDOFTRANSMISSION/1 -> Add1/1
  VERYSLOWCLK/1 -> Logical Operator1/1, ManualDeserializere/2(SLOWCLCK), CLKCNTERBOOTUP/2(CLK2CNT)
  2CLKDELAY/1 -> Logical Operator6/1
  2CLKDELAY2/1 -> BOOTUPCOMPLETE/1
  BOOTOFFSETT2/1 -> Relational Operator/2
  BOOTOFFSETT3/1 -> Relational Operator1/2, Add1/2, Add/2
  CLKCNTERBOOTUP/1(CNT) -> Relational Operator2/1, Relational Operator1/1, Relational Operator/1, OUTPUTCONTROLCONTINIOUS/1(CLKCNT)
  Constant/1 -> ManualDeserializere/3(DATA)
  Constant1/1 -> ManualDeserializere/5(14)
  Logical Operator/1 -> Logical Operator1/2, OUTPUTCONTROLCONTINIOUS/4(OPENCOM)
  Logical Operator1/1 -> Logical Operator2/1
  Logical Operator2/1 -> CLKOUT/1
  Logical Operator3/1 -> Logical Operator4/2, Logical Operator2/3
  Logical Operator4/1 -> ManualDeserializere/4(reset)
  Logical Operator5/1 -> 2CLKDELAY2/1
  Logical Operator6/1 -> DATAOUT/1
  ManualDeserializere/1(valin) -> 2CLKDELAY/1
  OUTPUTCONTROLCONTINIOUS/1(CLKOFF) -> Logical Operator5/1, Delay/1
  OUTPUTCONTROLCONTINIOUS/2(DATAINV) -> DATAINV/1
  Relational Operator/1 -> Logical Operator4/3, Logical Operator2/2
  Relational Operator1/1 -> Logical Operator3/2
  Relational Operator2/1 -> Logical Operator3/1
  TLOWOFFSET/1 -> Relational Operator2/2
  TmpGroundAtLogical Operator6Inport2/1 -> Logical Operator6/2
  OUTPUTCONTROLCONTINIOUS/3(RESETCNT) -> OUTPUTCONTROLCONTINIOUS_term2/1
  Add/1 -> OUTPUTCONTROLCONTINIOUS/2(CLKS2DATAFLOWCHG)
  Add1/1 -> OUTPUTCONTROLCONTINIOUS/3(CLK2ENDOFTRANSMISSION)
  Delay/1 -> Logical Operator/1

== system gm_UZ_EnDat_be4_segregation/UZ_ENDAT/ramselektor ==
  In1 : Inport  OutMin=0  OutMax=15  OutDataTypeStr=fixdt(0, 4, 0)  PortDimensions=1  SampleTime=1e-08  LockScale=on
  Trigger : Inport  Port=2  OutDataTypeStr=boolean  SampleTime=1e-08
  Delay : Subsystem
      settings: MinAlgLoopOccurrences=on
  Increment Stored Integer : Subsystem  mask(Stored Integer Value Increment){}
      mask help: Simulink:masks:StoredIntegerValueIncrement_MD
      mask Display: disp('Q++')
  Increment Stored Integer_out1bypassMux : MultiPortSwitch  DataPortOrder=Zero-based contiguous  Inputs=2  zeroidx=on  OutDataTypeStr=fixdt(0, 4, 0)  SampleTime=1e-08  SaturateOnIntegerOverflow=off  InputSameDT=off
  Trigger_delay : Delay  DelayLength=double(1)  InitialCondition=0
  Trigger_delay_Initial_Val : Constant  OutDataTypeStr=boolean  SampleTime=1e-08
  Trigger_delay_ctrl_const : Constant  OutDataTypeStr=boolean  SampleTime=1e-08
  Trigger_delay_ctrl_delay : Delay  DelayLength=double(1)  InitialCondition=0
  Trigger_delay_switch : Switch  Criteria=u2 ~= 0  Threshold=double(0)  OutDataTypeStr=boolean  SampleTime=1e-08  SaturateOnIntegerOverflow=off  InputSameDT=off
  Trigger_delayed_inverted_and_Trigger : Logic  AllPortsSameDT=off  OutDataTypeStr=boolean  SampleTime=1e-08
  not_Trigger_delayed : Logic  Operator=NOT  Inputs=1  AllPortsSameDT=off  OutDataTypeStr=boolean  SampleTime=1e-08
  out0_bypass : UnitDelay  InitialCondition="fi(0,0,4,0,\"hex\",\"0\")"  SampleTime=1e-08
  SEL : Outport  SampleTime=1e-08  InitialOutput=0
  wires:
  Trigger/1 -> Trigger_delayed_inverted_and_Trigger/2, Trigger_delay/1
  In1/1 -> Delay/1(in0)
  Increment Stored Integer_out1bypassMux/1 -> SEL/1, out0_bypass/1
  Trigger_delay_switch/1 -> not_Trigger_delayed/1
  not_Trigger_delayed/1 -> Trigger_delayed_inverted_and_Trigger/1
  Trigger_delayed_inverted_and_Trigger/1 -> Delay/Enable, Increment Stored Integer_out1bypassMux/1
  Trigger_delay/1 -> Trigger_delay_switch/1
  Trigger_delay_Initial_Val/1 -> Trigger_delay_switch/3
  Trigger_delay_ctrl_delay/1 -> Trigger_delay_switch/2
  Delay/1(out0) -> Increment Stored Integer/1(u)
  out0_bypass/1 -> Increment Stored Integer_out1bypassMux/2
  Increment Stored Integer/1(y) -> Increment Stored Integer_out1bypassMux/3
  Trigger_delay_ctrl_const/1 -> Trigger_delay_ctrl_delay/1

== system gm_UZ_EnDat_be4_segregation/UZ_ENDAT/16bitgather/Subsystem ==
  val : Inport  OutDataTypeStr=uint16  PortDimensions=1  SampleTime=1e-08
  set : Inport  Port=2  OutDataTypeStr=boolean  PortDimensions=1  SampleTime=1e-08
  Bit Set : simulink/Logic and Bit Operations/Bit Set  iBit=double(0)
  Switch : Switch  Criteria=u2 ~= 0  Threshold=double(0)  OutDataTypeStr=uint16  SampleTime=1e-08  SaturateOnIntegerOverflow=off  InputSameDT=off
  Out1 : Outport  SampleTime=1e-08
  wires:
  val/1 -> Switch/1, Bit Set/1
  set/1 -> Switch/2
  Bit Set/1 -> Switch/3
  Switch/1 -> Out1/1

== system gm_UZ_EnDat_be4_segregation/UZ_ENDAT/16bitgather/Subsystem1 ==
  val : Inport  OutDataTypeStr=uint16  PortDimensions=1  SampleTime=1e-08
  set : Inport  Port=2  OutDataTypeStr=boolean  PortDimensions=1  SampleTime=1e-08
  Bit Set : simulink/Logic and Bit Operations/Bit Set  iBit=double(1)
  Switch : Switch  Criteria=u2 ~= 0  Threshold=double(0)  OutDataTypeStr=uint16  SampleTime=1e-08  SaturateOnIntegerOverflow=off  InputSameDT=off
  Out1 : Outport  SampleTime=1e-08
  wires:
  val/1 -> Switch/1, Bit Set/1
  set/1 -> Switch/2
  Bit Set/1 -> Switch/3
  Switch/1 -> Out1/1

== system gm_UZ_EnDat_be4_segregation/UZ_ENDAT/16bitgather/Subsystem10 ==
  val : Inport  OutDataTypeStr=uint16  PortDimensions=1  SampleTime=1e-08
  set : Inport  Port=2  OutDataTypeStr=boolean  PortDimensions=1  SampleTime=1e-08
  Bit Set : simulink/Logic and Bit Operations/Bit Set  iBit=double(10)
  Switch : Switch  Criteria=u2 ~= 0  Threshold=double(0)  OutDataTypeStr=uint16  SampleTime=1e-08  SaturateOnIntegerOverflow=off  InputSameDT=off
  Out1 : Outport  SampleTime=1e-08
  wires:
  val/1 -> Switch/1, Bit Set/1
  set/1 -> Switch/2
  Bit Set/1 -> Switch/3
  Switch/1 -> Out1/1

== system gm_UZ_EnDat_be4_segregation/UZ_ENDAT/16bitgather/Subsystem11 ==
  val : Inport  OutDataTypeStr=uint16  PortDimensions=1  SampleTime=1e-08
  set : Inport  Port=2  OutDataTypeStr=boolean  PortDimensions=1  SampleTime=1e-08
  Bit Set : simulink/Logic and Bit Operations/Bit Set  iBit=double(11)
  Switch : Switch  Criteria=u2 ~= 0  Threshold=double(0)  OutDataTypeStr=uint16  SampleTime=1e-08  SaturateOnIntegerOverflow=off  InputSameDT=off
  Out1 : Outport  SampleTime=1e-08
  wires:
  val/1 -> Switch/1, Bit Set/1
  set/1 -> Switch/2
  Bit Set/1 -> Switch/3
  Switch/1 -> Out1/1

== system gm_UZ_EnDat_be4_segregation/UZ_ENDAT/16bitgather/Subsystem12 ==
  val : Inport  OutDataTypeStr=uint16  PortDimensions=1  SampleTime=1e-08
  set : Inport  Port=2  OutDataTypeStr=boolean  PortDimensions=1  SampleTime=1e-08
  Bit Set : simulink/Logic and Bit Operations/Bit Set  iBit=double(12)
  Switch : Switch  Criteria=u2 ~= 0  Threshold=double(0)  OutDataTypeStr=uint16  SampleTime=1e-08  SaturateOnIntegerOverflow=off  InputSameDT=off
  Out1 : Outport  SampleTime=1e-08
  wires:
  val/1 -> Switch/1, Bit Set/1
  set/1 -> Switch/2
  Bit Set/1 -> Switch/3
  Switch/1 -> Out1/1

== system gm_UZ_EnDat_be4_segregation/UZ_ENDAT/16bitgather/Subsystem13 ==
  val : Inport  OutDataTypeStr=uint16  PortDimensions=1  SampleTime=1e-08
  set : Inport  Port=2  OutDataTypeStr=boolean  PortDimensions=1  SampleTime=1e-08
  Bit Set : simulink/Logic and Bit Operations/Bit Set  iBit=double(13)
  Switch : Switch  Criteria=u2 ~= 0  Threshold=double(0)  OutDataTypeStr=uint16  SampleTime=1e-08  SaturateOnIntegerOverflow=off  InputSameDT=off
  Out1 : Outport  SampleTime=1e-08
  wires:
  val/1 -> Switch/1, Bit Set/1
  set/1 -> Switch/2
  Bit Set/1 -> Switch/3
  Switch/1 -> Out1/1

== system gm_UZ_EnDat_be4_segregation/UZ_ENDAT/16bitgather/Subsystem14 ==
  val : Inport  OutDataTypeStr=uint16  PortDimensions=1  SampleTime=1e-08
  set : Inport  Port=2  OutDataTypeStr=boolean  PortDimensions=1  SampleTime=1e-08
  Bit Set : simulink/Logic and Bit Operations/Bit Set  iBit=double(14)
  Switch : Switch  Criteria=u2 ~= 0  Threshold=double(0)  OutDataTypeStr=uint16  SampleTime=1e-08  SaturateOnIntegerOverflow=off  InputSameDT=off
  Out1 : Outport  SampleTime=1e-08
  wires:
  val/1 -> Switch/1, Bit Set/1
  set/1 -> Switch/2
  Bit Set/1 -> Switch/3
  Switch/1 -> Out1/1

== system gm_UZ_EnDat_be4_segregation/UZ_ENDAT/16bitgather/Subsystem15 ==
  val : Inport  OutDataTypeStr=uint16  PortDimensions=1  SampleTime=1e-08
  set : Inport  Port=2  OutDataTypeStr=boolean  PortDimensions=1  SampleTime=1e-08
  Bit Set : simulink/Logic and Bit Operations/Bit Set  iBit=double(13)
  Switch : Switch  Criteria=u2 ~= 0  Threshold=double(0)  OutDataTypeStr=uint16  SampleTime=1e-08  SaturateOnIntegerOverflow=off  InputSameDT=off
  Out1 : Outport  SampleTime=1e-08
  wires:
  val/1 -> Switch/1, Bit Set/1
  set/1 -> Switch/2
  Bit Set/1 -> Switch/3
  Switch/1 -> Out1/1

== system gm_UZ_EnDat_be4_segregation/UZ_ENDAT/16bitgather/Subsystem2 ==
  val : Inport  OutDataTypeStr=uint16  PortDimensions=1  SampleTime=1e-08
  set : Inport  Port=2  OutDataTypeStr=boolean  PortDimensions=1  SampleTime=1e-08
  Bit Set : simulink/Logic and Bit Operations/Bit Set  iBit=double(3)
  Switch : Switch  Criteria=u2 ~= 0  Threshold=double(0)  OutDataTypeStr=uint16  SampleTime=1e-08  SaturateOnIntegerOverflow=off  InputSameDT=off
  Out1 : Outport  SampleTime=1e-08
  wires:
  val/1 -> Switch/1, Bit Set/1
  set/1 -> Switch/2
  Bit Set/1 -> Switch/3
  Switch/1 -> Out1/1

== system gm_UZ_EnDat_be4_segregation/UZ_ENDAT/16bitgather/Subsystem3 ==
  val : Inport  OutDataTypeStr=uint16  PortDimensions=1  SampleTime=1e-08
  set : Inport  Port=2  OutDataTypeStr=boolean  PortDimensions=1  SampleTime=1e-08
  Bit Set : simulink/Logic and Bit Operations/Bit Set  iBit=double(4)
  Switch : Switch  Criteria=u2 ~= 0  Threshold=double(0)  OutDataTypeStr=uint16  SampleTime=1e-08  SaturateOnIntegerOverflow=off  InputSameDT=off
  Out1 : Outport  SampleTime=1e-08
  wires:
  val/1 -> Switch/1, Bit Set/1
  set/1 -> Switch/2
  Bit Set/1 -> Switch/3
  Switch/1 -> Out1/1

== system gm_UZ_EnDat_be4_segregation/UZ_ENDAT/16bitgather/Subsystem4 ==
  val : Inport  OutDataTypeStr=uint16  PortDimensions=1  SampleTime=1e-08
  set : Inport  Port=2  OutDataTypeStr=boolean  PortDimensions=1  SampleTime=1e-08
  Bit Set : simulink/Logic and Bit Operations/Bit Set  iBit=double(4)
  Switch : Switch  Criteria=u2 ~= 0  Threshold=double(0)  OutDataTypeStr=uint16  SampleTime=1e-08  SaturateOnIntegerOverflow=off  InputSameDT=off
  Out1 : Outport  SampleTime=1e-08
  wires:
  val/1 -> Switch/1, Bit Set/1
  set/1 -> Switch/2
  Bit Set/1 -> Switch/3
  Switch/1 -> Out1/1

== system gm_UZ_EnDat_be4_segregation/UZ_ENDAT/16bitgather/Subsystem5 ==
  val : Inport  OutDataTypeStr=uint16  PortDimensions=1  SampleTime=1e-08
  set : Inport  Port=2  OutDataTypeStr=boolean  PortDimensions=1  SampleTime=1e-08
  Bit Set : simulink/Logic and Bit Operations/Bit Set  iBit=double(5)
  Switch : Switch  Criteria=u2 ~= 0  Threshold=double(0)  OutDataTypeStr=uint16  SampleTime=1e-08  SaturateOnIntegerOverflow=off  InputSameDT=off
  Out1 : Outport  SampleTime=1e-08
  wires:
  val/1 -> Switch/1, Bit Set/1
  set/1 -> Switch/2
  Bit Set/1 -> Switch/3
  Switch/1 -> Out1/1

== system gm_UZ_EnDat_be4_segregation/UZ_ENDAT/16bitgather/Subsystem6 ==
  val : Inport  OutDataTypeStr=uint16  PortDimensions=1  SampleTime=1e-08
  set : Inport  Port=2  OutDataTypeStr=boolean  PortDimensions=1  SampleTime=1e-08
  Bit Set : simulink/Logic and Bit Operations/Bit Set  iBit=double(6)
  Switch : Switch  Criteria=u2 ~= 0  Threshold=double(0)  OutDataTypeStr=uint16  SampleTime=1e-08  SaturateOnIntegerOverflow=off  InputSameDT=off
  Out1 : Outport  SampleTime=1e-08
  wires:
  val/1 -> Switch/1, Bit Set/1
  set/1 -> Switch/2
  Bit Set/1 -> Switch/3
  Switch/1 -> Out1/1

== system gm_UZ_EnDat_be4_segregation/UZ_ENDAT/16bitgather/Subsystem7 ==
  val : Inport  OutDataTypeStr=uint16  PortDimensions=1  SampleTime=1e-08
  set : Inport  Port=2  OutDataTypeStr=boolean  PortDimensions=1  SampleTime=1e-08
  Bit Set : simulink/Logic and Bit Operations/Bit Set  iBit=double(7)
  Switch : Switch  Criteria=u2 ~= 0  Threshold=double(0)  OutDataTypeStr=uint16  SampleTime=1e-08  SaturateOnIntegerOverflow=off  InputSameDT=off
  Out1 : Outport  SampleTime=1e-08
  wires:
  val/1 -> Switch/1, Bit Set/1
  set/1 -> Switch/2
  Bit Set/1 -> Switch/3
  Switch/1 -> Out1/1

== system gm_UZ_EnDat_be4_segregation/UZ_ENDAT/16bitgather/Subsystem8 ==
  val : Inport  OutDataTypeStr=uint16  PortDimensions=1  SampleTime=1e-08
  set : Inport  Port=2  OutDataTypeStr=boolean  PortDimensions=1  SampleTime=1e-08
  Bit Set : simulink/Logic and Bit Operations/Bit Set  iBit=double(8)
  Switch : Switch  Criteria=u2 ~= 0  Threshold=double(0)  OutDataTypeStr=uint16  SampleTime=1e-08  SaturateOnIntegerOverflow=off  InputSameDT=off
  Out1 : Outport  SampleTime=1e-08
  wires:
  val/1 -> Switch/1, Bit Set/1
  set/1 -> Switch/2
  Bit Set/1 -> Switch/3
  Switch/1 -> Out1/1

== system gm_UZ_EnDat_be4_segregation/UZ_ENDAT/16bitgather/Subsystem9 ==
  val : Inport  OutDataTypeStr=uint16  PortDimensions=1  SampleTime=1e-08
  set : Inport  Port=2  OutDataTypeStr=boolean  PortDimensions=1  SampleTime=1e-08
  Bit Set : simulink/Logic and Bit Operations/Bit Set  iBit=double(9)
  Switch : Switch  Criteria=u2 ~= 0  Threshold=double(0)  OutDataTypeStr=uint16  SampleTime=1e-08  SaturateOnIntegerOverflow=off  InputSameDT=off
  Out1 : Outport  SampleTime=1e-08
  wires:
  val/1 -> Switch/1, Bit Set/1
  set/1 -> Switch/2
  Bit Set/1 -> Switch/3
  Switch/1 -> Out1/1
